simulink model "LQR_single"  (R2019a)
settings: Solver=FixedStepAuto  StartTime=0.0  StopTime=24.9  FixedStep=0.0001  RelTol=1e-3
values from neighbouring files (symbols this model uses):
  Cf = 30989    [LQR_Setup.m]
  Cr = 50154    [LQR_Setup.m]
  Iz = 111.8    [LQR_Setup.m]
  K1l = K(1,1)    [LQR_Setup.m]
  K2l = K(1,2)    [LQR_Setup.m]
  K3l = K(1,3)    [LQR_Setup.m]
  lf = 0.783    [LQR_Setup.m]
  lr = 0.752    [LQR_Setup.m]
  m = 245    [LQR_Setup.m]
undefined symbols (not defined in the file or in its folder): DiscIntNeverNeededParam
libraries: dspsrcs4 x4
settings Model: Creator=Johan PC  LastModifiedBy=Johan PC
settings DataIOCC: ReturnWorkspaceOutputs=off
settings DebuggingCC: ArithmeticOperatorsInVariantConditions=warning

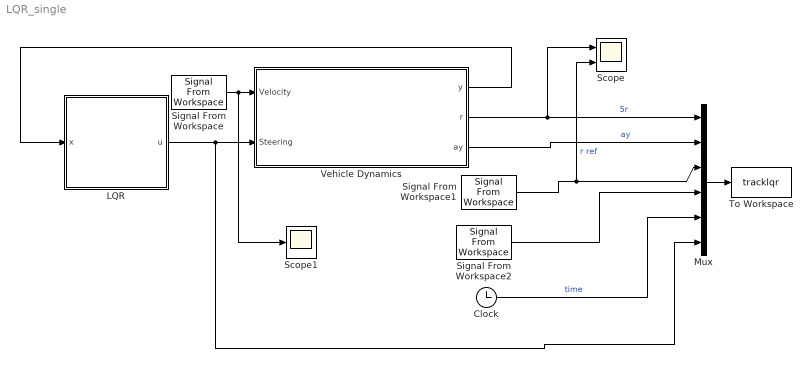
== system LQR_single ==
  Clock : Clock
  LQR : Subsystem
  Mux : Mux  Inputs=6
  Scope : Scope  NumInputPorts=2
  Scope1 : Scope
  Signal From Workspace : dspsrcs4/Signal From Workspace  X=Velocityi  Ts=0.12  nsamps=1  OutputAfterFinalValue=Setting to zero  ignoreOrWarnInputAndFrameLengths=off  OutputFrames=off
  Signal From Workspace1 : dspsrcs4/Signal From Workspace  X=Yawrate  Ts=0.12  nsamps=1  OutputAfterFinalValue=Setting to zero  ignoreOrWarnInputAndFrameLengths=off  OutputFrames=off
  Signal From Workspace2 : dspsrcs4/Signal From Workspace  X=Lat_Acc  Ts=0.12  nsamps=1  OutputAfterFinalValue=Setting to zero  ignoreOrWarnInputAndFrameLengths=off  OutputFrames=off
  To Workspace : ToWorkspace  VariableName=tracklqr  SampleTime=-1
      settings: Save2DSignal=2-D array (concatenate along first dimension)
  Vehicle Dynamics : Subsystem
  wires:
  Vehicle Dynamics/1("y ") -> LQR/1(x)
  LQR/1(u) -> Mux/6, Vehicle Dynamics/2(Steering)
  Vehicle Dynamics/2("r ") -> Scope/1, Mux/1  "5r"
  Vehicle Dynamics/3(ay) -> Mux/2  "ay"
  Mux/1 -> To Workspace/1
  Signal From Workspace/1 -> Scope1/1, Vehicle Dynamics/1(Velocity)
  Signal From Workspace1/1 -> Scope/2, Mux/3  "r ref"
  Signal From Workspace2/1 -> Mux/4
  Clock/1 -> Mux/5  "time"

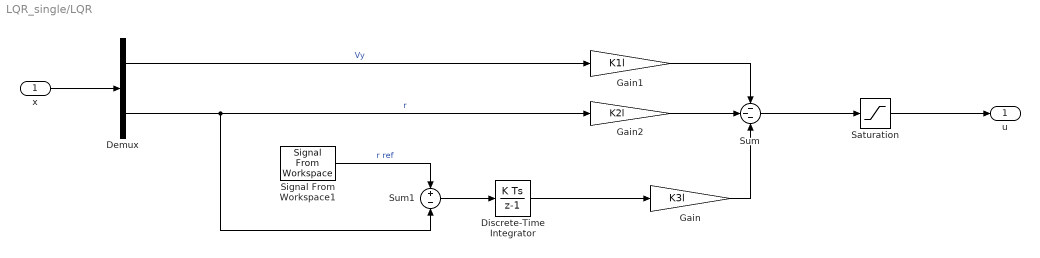
== system LQR_single/LQR ==
  x : Inport
  Demux : Demux  Outputs=2
  Discrete-Time Integrator : DiscreteIntegrator  SampleTime=0.001  ICPrevOutput=DiscIntNeverNeededParam  ICPrevScaledInput=DiscIntNeverNeededParam
  Gain : Gain  Gain=K3l
  Gain1 : Gain  Gain=K1l
  Gain2 : Gain  Gain=K2l
  Saturation : Saturate  UpperLimit=0.45  LowerLimit=-0.45
  Signal From Workspace1 : dspsrcs4/Signal From Workspace  X=Yawrate  Ts=0.12  nsamps=1  OutputAfterFinalValue=Setting to zero  ignoreOrWarnInputAndFrameLengths=off  OutputFrames=off
  Sum : Sum  Inputs=---
  Sum1 : Sum  Inputs=+-
  u : Outport
  wires:
  Discrete-Time Integrator/1 -> Gain/1
  Gain/1 -> Sum/3
  x/1 -> Demux/1
  Demux/1 -> Gain1/1  "Vy"
  Demux/2 -> Gain2/1, Sum1/2  "r"
  Gain1/1 -> Sum/1
  Gain2/1 -> Sum/2
  Sum/1 -> Saturation/1
  Sum1/1 -> Discrete-Time Integrator/1
  Signal From Workspace1/1 -> Sum1/1  "r ref"
  Saturation/1 -> u/1

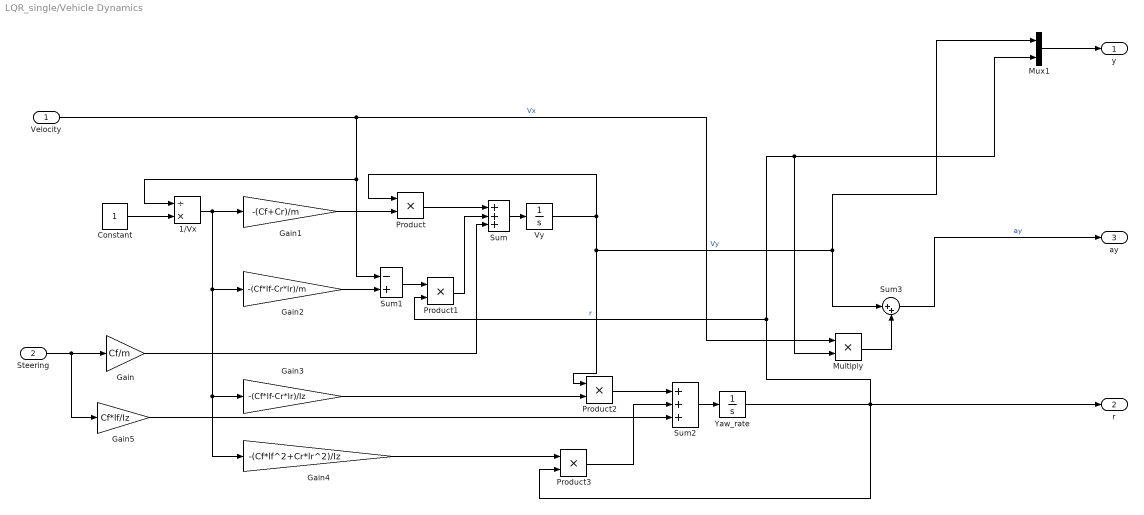
== system LQR_single/Vehicle Dynamics ==
  Velocity : Inport
  Steering : Inport  Port=2
  1/Vx : Product  Inputs=/*
  Constant : Constant
  Gain : Gain  Gain=Cf/m
  Gain1 : Gain  Gain=-(Cf+Cr)/m
  Gain2 : Gain  Gain=-(Cf*lf-Cr*lr)/m
  Gain3 : Gain  Gain=-(Cf*lf-Cr*lr)/Iz
  Gain4 : Gain  Gain=-(Cf*lf^2+Cr*lr^2)/Iz
  Gain5 : Gain  Gain=Cf*lf/Iz
  Multiply : Product
  Mux1 : Mux  Inputs=2
  Product{,1..3} (4 alike) : Product
  Sum : Sum  Inputs=+++
  Sum1 : Sum  Inputs=-+
  Sum2 : Sum  Inputs=+++
  Sum3 : Sum  Inputs=|++
  Vy : Integrator
  "Yaw_rate " : Integrator
  "y " : Outport
  "r " : Outport  Port=2
  ay : Outport  Port=3
  wires:
  Sum2/1 -> "Yaw_rate "/1
  Gain2/1 -> Sum1/2
  Gain4/1 -> Product3/1
  Constant/1 -> 1/Vx/2
  Gain3/1 -> Product2/2
  1/Vx/1 -> Gain4/1, Gain3/1, Gain2/1, Gain1/1
  Product2/1 -> Sum2/1
  Product3/1 -> Sum2/2
  Gain5/1 -> Sum2/3
  Sum1/1 -> Product1/1
  "Yaw_rate "/1 -> Multiply/2, Mux1/2, Product1/2, "r "/1, Product3/2  "r"
  Gain/1 -> Sum/3
  Steering/1 -> Gain/1, Gain5/1
  Gain1/1 -> Product/2
  Product/1 -> Sum/1
  Vy/1 -> Mux1/1, Sum3/1, Product2/1, Product/1  "Vy"
  Sum/1 -> Vy/1
  Velocity/1 -> Multiply/1, 1/Vx/1, Sum1/1  "Vx"
  Product1/1 -> Sum/2
  Multiply/1 -> Sum3/2
  Sum3/1 -> ay/1  "ay"
  Mux1/1 -> "y "/1
